simulink model "Final_2022"  (R2016a)
settings: Solver=VariableStepAuto  StartTime=0.0  StopTime=10.0  RelTol=1e-3
libraries: simulink x2
settings Model: Creator=alber  LastModifiedBy=alber

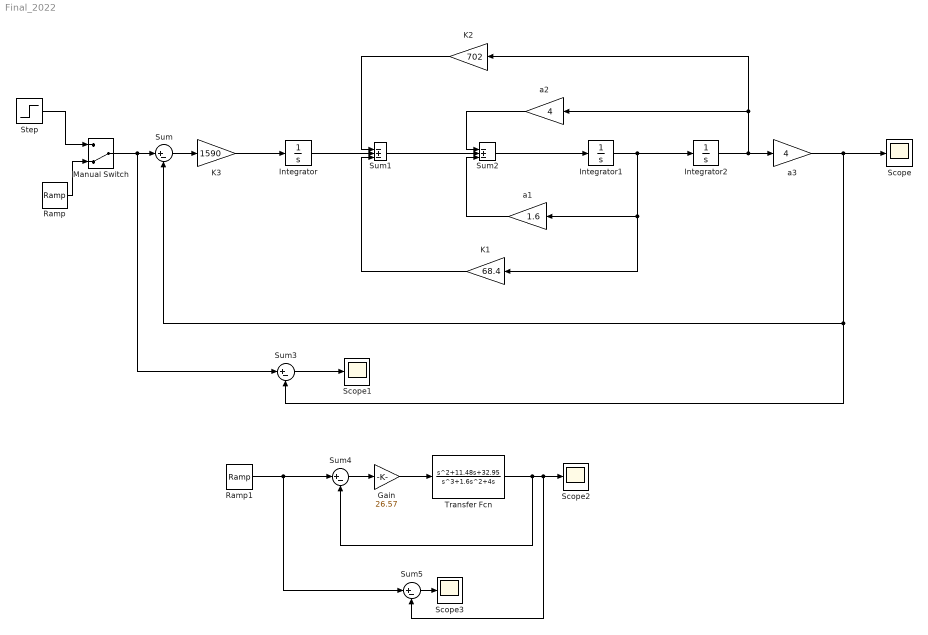
== system Final_2022 ==
  Gain : Gain  Gain=26.57
  Integrator : Integrator
  Integrator1 : Integrator
  Integrator2 : Integrator
  K1 : Gain  Gain=68.4
  K2 : Gain  Gain=702
  K3 : Gain  Gain=1590
  Manual Switch : ManualSwitch  CurrentSetting=0
  Ramp : simulink/Sources/Ramp  slope=1  start=0  X0=0
  Ramp1 : simulink/Sources/Ramp  slope=1  start=0  X0=0
  Scope{,1..3} (4 alike) : Scope
  Step : Step  SampleTime=0
  Sum{,3..5} (4 alike) : Sum  Inputs=|+-
  Sum1 : Sum  Inputs=|-+-
  Sum2 : Sum  Inputs=|-+-
  Transfer Fcn : TransferFcn  Numerator=[1 11.48 32.95]  Denominator=[1 1.6 4 0]
  a1 : Gain  Gain=1.6
  a2 : Gain  Gain=4
  a3 : Gain  Gain=4
  wires:
  Sum/1 -> K3/1
  K3/1 -> Integrator/1
  Integrator/1 -> Sum1/2
  Sum1/1 -> Sum2/2
  Sum2/1 -> Integrator1/1
  Integrator1/1 -> K1/1, a1/1, Integrator2/1
  a1/1 -> Sum2/3
  K1/1 -> Sum1/3
  Integrator2/1 -> K2/1, a2/1, a3/1
  a3/1 -> Sum/2, Sum3/2, Scope/1
  a2/1 -> Sum2/1
  K2/1 -> Sum1/1
  Ramp1/1 -> Sum4/1, Sum5/1
  Transfer Fcn/1 -> Sum4/2, Sum5/2, Scope2/1
  Sum5/1 -> Scope3/1
  Sum4/1 -> Gain/1
  Gain/1 -> Transfer Fcn/1
  Manual Switch/1 -> Sum3/1, Sum/1
  Ramp/1 -> Manual Switch/2
  Step/1 -> Manual Switch/1
  Sum3/1 -> Scope1/1
